simulink model "udp_send_agg"  (R2021b)
settings: Solver=VariableStepAuto  StartTime=0.0  StopTime=10.0  RelTol=1e-3
libraries: slrealtimeutilitieslib x4, slrealtimeiplib x1
settings Model: Creator=Amyang  LastModifiedBy=Amyang

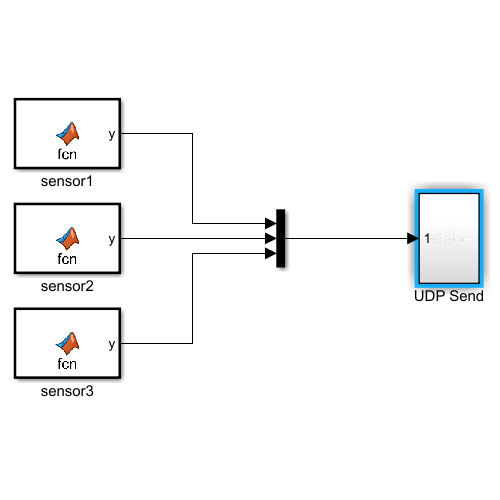
[thumbnail: Simulink's stored preview of the top-level diagram]
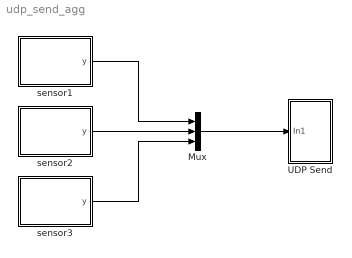
== system udp_send_agg ==
  Mux : Mux  Inputs=3
  UDP Send : Subsystem
  sensor1 : MATLAB Function  TreatAsAtomicUnit=on
  sensor2 : MATLAB Function  TreatAsAtomicUnit=on
  sensor3 : MATLAB Function  TreatAsAtomicUnit=on
  wires:
  sensor1/1(y) -> Mux/1
  sensor2/1(y) -> Mux/2
  sensor3/1(y) -> Mux/3
  Mux/1 -> UDP Send/1(In1)

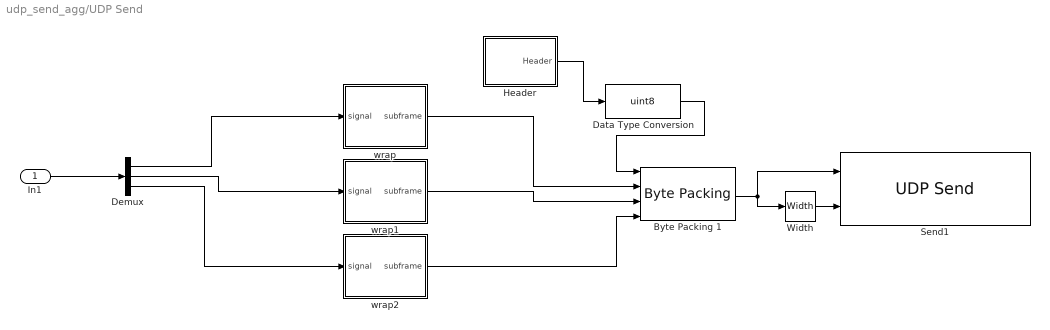
== system udp_send_agg/UDP Send ==
  In1 : Inport
  Byte Packing 1 : slrealtimeutilitieslib/Byte Packing  MaskPackedDataType=uint8  MaskUnpackedDataTypes={'uint8','uint8','uint8','uint8'}  MaskAlignment=1
  Data Type Conversion : DataTypeConversion  OutDataTypeStr=uint8
  Demux : Demux  Outputs=3
  Header : MATLAB Function  TreatAsAtomicUnit=on
  Send1 : slrealtimeiplib/UDP Send  useHostTargetConn=on  toAddress=192.168.1.4  toPort=10001  sampleTime=1  localPort=-1
      settings: SourceProductBaseCode=XP
  Width : Width
  wrap : Subsystem
  wrap1 : Subsystem
  wrap2 : Subsystem
  wires:
  Demux/1 -> wrap/1(signal)
  wrap2/1(subframe) -> Byte Packing 1/4
  Demux/2 -> wrap1/1(signal)
  Byte Packing 1/1 -> Send1/1, Width/1
  wrap1/1(subframe) -> Byte Packing 1/3
  Width/1 -> Send1/2
  wrap/1(subframe) -> Byte Packing 1/2
  Demux/3 -> wrap2/1(signal)
  In1/1 -> Demux/1
  Header/1(Header) -> Data Type Conversion/1
  Data Type Conversion/1 -> Byte Packing 1/1

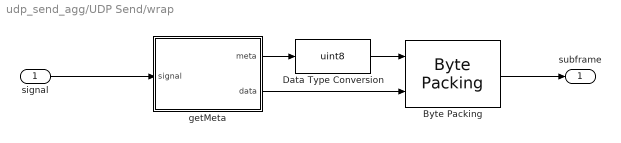
== system udp_send_agg/UDP Send/wrap ==
  signal : Inport
  "Byte Packing " : slrealtimeutilitieslib/Byte Packing  MaskPackedDataType=uint8  MaskUnpackedDataTypes={'uint8','double'}  MaskAlignment=1
  Data Type Conversion : DataTypeConversion  OutDataTypeStr=uint8
  getMeta : MATLAB Function  TreatAsAtomicUnit=on
  subframe : Outport
  wires:
  getMeta/1(meta) -> Data Type Conversion/1
  signal/1 -> getMeta/1(signal)
  Data Type Conversion/1 -> "Byte Packing "/1
  getMeta/2(data) -> "Byte Packing "/2
  "Byte Packing "/1 -> subframe/1

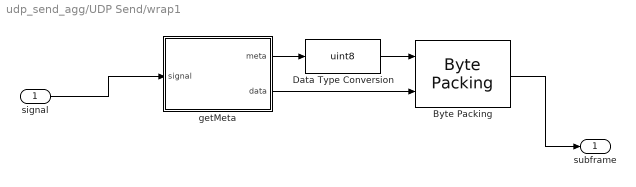
== system udp_send_agg/UDP Send/wrap1 ==
  signal : Inport
  "Byte Packing " : slrealtimeutilitieslib/Byte Packing  MaskPackedDataType=uint8  MaskUnpackedDataTypes={'uint8','double'}  MaskAlignment=1
  Data Type Conversion : DataTypeConversion  OutDataTypeStr=uint8
  getMeta : MATLAB Function  TreatAsAtomicUnit=on
  subframe : Outport
  wires:
  getMeta/1(meta) -> Data Type Conversion/1
  signal/1 -> getMeta/1(signal)
  Data Type Conversion/1 -> "Byte Packing "/1
  getMeta/2(data) -> "Byte Packing "/2
  "Byte Packing "/1 -> subframe/1

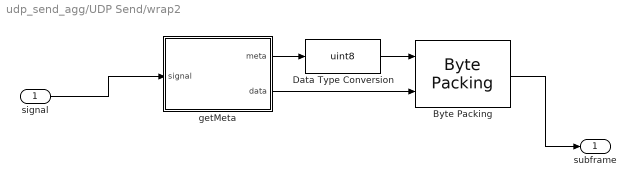
== system udp_send_agg/UDP Send/wrap2 ==
  signal : Inport
  "Byte Packing " : slrealtimeutilitieslib/Byte Packing  MaskPackedDataType=uint8  MaskUnpackedDataTypes={'uint8','double'}  MaskAlignment=1
  Data Type Conversion : DataTypeConversion  OutDataTypeStr=uint8
  getMeta : MATLAB Function  TreatAsAtomicUnit=on
  subframe : Outport
  wires:
  getMeta/1(meta) -> Data Type Conversion/1
  signal/1 -> getMeta/1(signal)
  Data Type Conversion/1 -> "Byte Packing "/1
  getMeta/2(data) -> "Byte Packing "/2
  "Byte Packing "/1 -> subframe/1

== matlab function udp_send_agg/sensor2 ==
  data: y output
function y = fcn()

y = [4,5,6];

== matlab function udp_send_agg/sensor1 ==
  data: y output
function y = fcn()

y = [1,2,3];

== matlab function udp_send_agg/sensor3 ==
  data: y output
function y = fcn()

y = [7,8,9];

== matlab function udp_send_agg/UDP Send/wrap1/getMeta ==
  data: meta output; signal input; data output
function [meta,data]=get_meta(signal) % type, size, length

[row, col]=size(signal);

len = row*col;
% to-do, other fileds
meta=[row, col, len];
data = signal;

== matlab function udp_send_agg/UDP Send/wrap2/getMeta ==
  data: meta output; signal input; data output
function [meta,data]=get_meta(signal) % type, size, length

[row, col]=size(signal);

len = row*col;
% to-do, other fileds
meta=[row, col, len];
data = signal;

== matlab function udp_send_agg/UDP Send/Header ==
  data: Header output
function Header = Header()
src = 111;
dst = 2;
subframes_N = 3; % configure manually
Header = [src, dst,subframes_N];

== matlab function udp_send_agg/UDP Send/wrap/getMeta ==
  data: meta output; signal input; data output
function [meta,data]=get_meta(signal) % type, size, length

[row, col]=size(signal);

len = row*col;
% to-do, other fileds
meta=[row, col, len];
data = signal;
